simulink library "FVT_lib"  (R2021b)
settings: Solver=VariableStepAuto  StartTime=0.0  StopTime=10.0  RelTol=1e-3
undefined symbols (not defined in the file): C_TASK_5MS_S, CANFDArray, ENUM_FAULTSTATE_FAIL, ENUM_FAULTSTATE_INDETERMINATE, ENUM_FAULTSTATE_PASS, EPSILON, FALSE, KHAL_CounterMAX_enum, KHAL_CounterMAXE2E_enum, LINArray, ONE_INT, TRUE, UNKNOWN, XX2KXX, ZERO_FLOAT, ZERO_INT
libraries: hdlsllib x41, simulink x24, hcu_lib x7
(part 3 of 3)

== system FVT_lib/hal/DDM_ESC5_CS&RC_Comparison/CRC8_Compare/DetectChange2 ==
  cnt : Inport
  Constant : Constant  OutDataTypeStr=boolean
  Data Type Conversion3 : DataTypeConversion  OutDataTypeStr=uint8
  Delay : Delay  DelayLength=1  InitialCondition=0
  Delay1 : Delay  DelayLength=1  InitialCondition=0
  Logical Operator : Logic  AllPortsSameDT=off  OutDataTypeStr=boolean
  Relational Operator : RelationalOperator  Operator=~=  OutDataTypeStr=boolean  RndMeth=Simplest
  InValid : Outport
  wires:
  Logical Operator/1 -> InValid/1
  Relational Operator/1 -> Logical Operator/1
  Delay1/1 -> Logical Operator/2
  Constant/1 -> Delay1/1
  cnt/1 -> Delay/1, Relational Operator/1
  Delay/1 -> Data Type Conversion3/1
  Data Type Conversion3/1 -> Relational Operator/2

== system FVT_lib/hal/DDM_ESC5_CS&RC_Comparison/CRC8_Compare/Subsystem ==
  RC : Inport
  RC_delay : Inport  Port=2
  Enable : EnablePort
  Equal1 : RelationalOperator  Operator===  OutDataTypeStr=boolean  RndMeth=Simplest
  RCErr : Outport
  wires:
  RC_delay/1 -> Equal1/2
  Equal1/1 -> RCErr/1
  RC/1 -> Equal1/1

== system FVT_lib/hal/DDM_ESC5_CS&RC_Comparison/CRC8_Compare/Timer ==
  note: /* output signal type is single */
  trigger : Inport
  reset : Inport  Port=2
  Ts : Inport  Port=3
  max_time : Inport  Port=4
  Constant1 : Constant  Value=ZERO_FLOAT  OutDataTypeStr=single
  GreaterThan : RelationalOperator  Operator=<=  OutDataTypeStr=boolean  RndMeth=Simplest
  Subtract2 : Sum
  Switch : Switch  Criteria=u2 > Threshold
  Switch1 : Switch  Criteria=u2 ~= 0
      settings: AttributesFormatString=<%<Criteria>>
  Switch2 : Switch  Criteria=u2 ~= 0
      settings: AttributesFormatString=<%<Criteria>>
  Unit Delay1 : UnitDelay  SampleTime=-1  HasFrameUpgradeWarning=on
      settings: AttributesFormatString=<initial = %<X0>>
  time : Outport
  wires:
  GreaterThan/1 -> Switch/2
  Subtract2/1 -> Switch2/1
  trigger/1 -> Switch2/2
  reset/1 -> Switch1/2
  Constant1/1 -> Switch1/1
  Switch1/1 -> Switch2/3
  Ts/1 -> Subtract2/2
  Switch2/1 -> GreaterThan/2, Switch/3
  Switch/1 -> Unit Delay1/1, time/1
  Unit Delay1/1 -> Switch1/3, [last_time]
  max_time/1 -> GreaterThan/1, Switch/1
  [last_time] -> Subtract2/1

== system FVT_lib/hal/DDM_ESC5_CS&RC_Comparison/CRC8_IfAction_Rx/If Action Subsystem ==
  Raw : Inport
  Action Port : ActionPort
  CRC8_Caculation : Subsystem
      mask help: MeasumentTrigerEvent
      mask Display: fprintf('CRC8');
  CRC8_Result : Outport
  wires:
  CRC8_Caculation/1(CRCout) -> CRC8_Result/1
  Raw/1 -> CRC8_Caculation/1(MsgData)

== system FVT_lib/hal/DDM_ESC5_CS&RC_Comparison/CRC8_IfAction_Rx/If Action Subsystem1 ==
  CAN_E2E_ID1 : Inport
  CAN_E2E_ID2 : Inport  Port=2
  Raw : Inport  Port=3
  Action Port : ActionPort
  CRC8_E2EProfile1 : Subsystem
      mask help: MeasumentTrigerEvent
      mask Display: fprintf('CRC8_E2EProfile1');
  Mux2 : Mux  Inputs=3
  CRC8_E2EResult : Outport
  wires:
  Mux2/1 -> CRC8_E2EProfile1/1(MsgData)
  CAN_E2E_ID1/1 -> Mux2/1
  CAN_E2E_ID2/1 -> Mux2/2
  Raw/1 -> Mux2/3
  CRC8_E2EProfile1/1(CRCout) -> CRC8_E2EResult/1

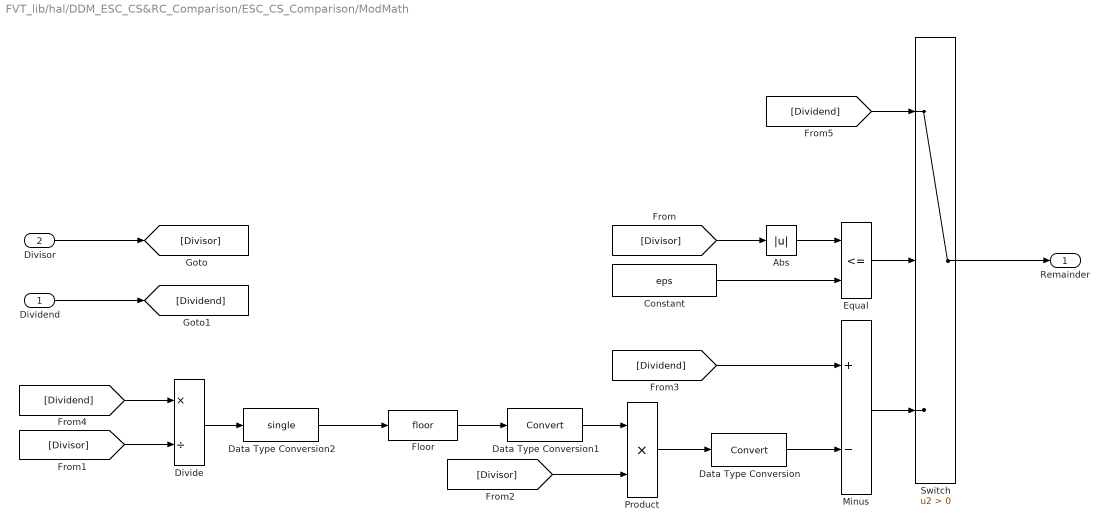
== system FVT_lib/hal/DDM_ESC_CS&RC_Comparison/ESC_CS_Comparison/ModMath ==
  Dividend : Inport
  Divisor : Inport  Port=2
  Abs : Abs
  Constant : Constant  Value=eps
  Data Type Conversion : DataTypeConversion
  Data Type Conversion1 : DataTypeConversion
  Data Type Conversion2 : DataTypeConversion  OutDataTypeStr=single
  Divide : Product  Inputs=*/
  Equal : RelationalOperator  Operator=<=  OutDataTypeStr=boolean  RndMeth=Simplest
  Floor : Rounding
  Minus : Sum  Inputs=+-
  Product : Product
  Switch : Switch  Criteria=u2 > Threshold
  Remainder : Outport
  wires:
  Divisor/1 -> [Divisor]
  Equal/1 -> Switch/2
  Constant/1 -> Equal/2
  [Dividend] -> Divide/1
  Switch/1 -> Remainder/1
  [Dividend] -> Switch/1
  Minus/1 -> Switch/3
  Data Type Conversion2/1 -> Floor/1
  Data Type Conversion/1 -> Minus/2
  [Dividend] -> Minus/1
  Dividend/1 -> [Dividend]
  Floor/1 -> Data Type Conversion1/1
  Data Type Conversion1/1 -> Product/1
  [Divisor] -> Divide/2
  Abs/1 -> Equal/1
  [Divisor] -> Product/2
  Divide/1 -> Data Type Conversion2/1
  Product/1 -> Data Type Conversion/1
  [Divisor] -> Abs/1

== system FVT_lib/hal/DDM_ESC_CS&RC_Comparison/RC_Compare/Counter ==
  note: /* Max Value of counter is 65535 */
  trigger : Inport
  reset : Inport  Port=2
  max_count : Inport  Port=3
  Constant1 : Constant  Value=ZERO_INT  OutDataTypeStr=uint16
  Constant2 : Constant  Value=uint16(1)  OutDataTypeStr=uint16
  Data Type Conversion : DataTypeConversion  OutDataTypeStr=uint16
  MinMax : MinMax  Inputs=2
  Saturation : Saturate  UpperLimit=65535  LowerLimit=0
      settings: AttributesFormatString=<upper = %<UpperLimit>>\n<lower = %<LowerLimit>>
  Subtract2 : Sum
  Switch1 : Switch  Criteria=u2 ~= 0
      settings: AttributesFormatString=<%<Criteria>>
  Switch2 : Switch  Criteria=u2 ~= 0
      settings: AttributesFormatString=<%<Criteria>>
  Unit Delay1 : UnitDelay  SampleTime=-1  HasFrameUpgradeWarning=on
      settings: AttributesFormatString=<initial = %<X0>>
  count : Outport
  wires:
  Data Type Conversion/1 -> Unit Delay1/1, count/1
  Subtract2/1 -> Switch2/1
  trigger/1 -> Switch2/2
  Switch2/1 -> Switch1/3
  Switch1/1 -> MinMax/2
  reset/1 -> Switch1/2
  Constant1/1 -> Switch1/1
  Constant2/1 -> Subtract2/2
  MinMax/1 -> Data Type Conversion/1
  Unit Delay1/1 -> [last_count], Switch2/3
  max_count/1 -> Saturation/1
  [last_count] -> Subtract2/1
  Saturation/1 -> MinMax/1

== system FVT_lib/hal/DDM_ESC_CS&RC_Comparison/RC_Compare/DetectChange2 ==
  cnt : Inport
  Constant : Constant  OutDataTypeStr=boolean
  Data Type Conversion3 : DataTypeConversion  OutDataTypeStr=uint8
  Delay : Delay  DelayLength=1  InitialCondition=0
  Delay1 : Delay  DelayLength=1  InitialCondition=0
  Logical Operator : Logic  AllPortsSameDT=off  OutDataTypeStr=boolean
  Relational Operator : RelationalOperator  Operator=~=  OutDataTypeStr=boolean  RndMeth=Simplest
  InValid : Outport
  wires:
  Logical Operator/1 -> InValid/1
  Relational Operator/1 -> Logical Operator/1
  Delay1/1 -> Logical Operator/2
  Constant/1 -> Delay1/1
  cnt/1 -> Delay/1, Relational Operator/1
  Delay/1 -> Data Type Conversion3/1
  Data Type Conversion3/1 -> Relational Operator/2

== system FVT_lib/hal/DDM_ESC_CS&RC_Comparison/RC_Compare/Subsystem ==
  RC : Inport
  RC_delay : Inport  Port=2
  Enable : EnablePort
  Equal1 : RelationalOperator  Operator===  OutDataTypeStr=boolean  RndMeth=Simplest
  RCErr : Outport
  wires:
  RC_delay/1 -> Equal1/2
  Equal1/1 -> RCErr/1
  RC/1 -> Equal1/1

== system FVT_lib/hal/DDM_ESC_CS&RC_Comparison/RC_Compare/Timer ==
  note: /* output signal type is single */
  trigger : Inport
  reset : Inport  Port=2
  Ts : Inport  Port=3
  max_time : Inport  Port=4
  Constant1 : Constant  Value=ZERO_FLOAT  OutDataTypeStr=single
  GreaterThan : RelationalOperator  Operator=<=  OutDataTypeStr=boolean  RndMeth=Simplest
  Subtract2 : Sum
  Switch : Switch  Criteria=u2 > Threshold
  Switch1 : Switch  Criteria=u2 ~= 0
      settings: AttributesFormatString=<%<Criteria>>
  Switch2 : Switch  Criteria=u2 ~= 0
      settings: AttributesFormatString=<%<Criteria>>
  Unit Delay1 : UnitDelay  SampleTime=-1  HasFrameUpgradeWarning=on
      settings: AttributesFormatString=<initial = %<X0>>
  time : Outport
  wires:
  GreaterThan/1 -> Switch/2
  Subtract2/1 -> Switch2/1
  trigger/1 -> Switch2/2
  reset/1 -> Switch1/2
  Constant1/1 -> Switch1/1
  Switch1/1 -> Switch2/3
  Ts/1 -> Subtract2/2
  Switch2/1 -> GreaterThan/2, Switch/3
  Switch/1 -> Unit Delay1/1, time/1
  Unit Delay1/1 -> Switch1/3, [last_time]
  max_time/1 -> GreaterThan/1, Switch/1
  [last_time] -> Subtract2/1

== system FVT_lib/inp/CAN_Msg_Validity_Process_template/CAN_Msg_Validity_Process/override_signal_m2  ==
  note: ONLY ONE ovrdflg (Service_ovrdflg and Cal_ovrdflg) can be valid
      | Set the priority of Service_ovrdflg higher than Cal_ovrdflg
      | In this way, the Cal_ovrd can be automatically disabled in production
  signal_raw : Inport
  cal_ovrdflg : Inport  Port=2
  cal_ovrdval : Inport  Port=3
  Switch1 : Switch  Criteria=u2 ~= 0  Threshold=0.5
  signal : Outport
  wires:
  cal_ovrdflg/1 -> Switch1/2  "cal_ovrdflg"
  cal_ovrdval/1 -> Switch1/1  "cal_ovrdval"
  signal_raw/1 -> Switch1/3  "signal_raw"
  Switch1/1 -> signal/1

== system FVT_lib/inp/ad_signal_template/ad_signal_process/override_signal_m2  ==
  note: ONLY ONE ovrdflg (Service_ovrdflg and Cal_ovrdflg) can be valid
      | Set the priority of Service_ovrdflg higher than Cal_ovrdflg
      | In this way, the Cal_ovrd can be automatically disabled in production
  note: When either service_ovrdflg or cal_ovrdflg is true, signal_valid_flg is set as TRUE
  signal_valid_flg_raw : Inport
  signal_raw : Inport  Port=2
  service_ovrdflg : Inport  Port=3
  service_ovrdval : Inport  Port=4
  cal_ovrdflg : Inport  Port=5
  cal_ovrdval : Inport  Port=6
  Data Type Duplicate : DataTypeDuplicate  NumInputPorts=5
  Logical Operator : Logic  Operator=OR  AllPortsSameDT=off  OutDataTypeStr=boolean
  Switch : Switch  Criteria=u2 ~= 0  Threshold=0.5
  Switch1 : Switch  Criteria=u2 ~= 0  Threshold=0.5
  Switch2 : Switch  Criteria=u2 ~= 0  Threshold=0.5
  True : Constant  Value=TRUE  OutDataTypeStr=boolean
  signal : Outport
  signal_valid_flg : Outport  Port=2
  wires:
  [cal_ovrdflg] -> Logical Operator/2
  [service_ovrdflg] -> Logical Operator/1
  Switch/1 -> Data Type Duplicate/5, signal/1  "signal"
  service_ovrdflg/1 -> [service_ovrdflg], Switch/2  "service_ovrdflg"
  cal_ovrdflg/1 -> [cal_ovrdflg], Switch1/2  "cal_ovrdflg"
  service_ovrdval/1 -> Data Type Duplicate/3, Switch/1  "service_ovrdval"
  cal_ovrdval/1 -> Data Type Duplicate/2, Switch1/1  "cal_ovrdval"
  signal_raw/1 -> Data Type Duplicate/1, Switch1/3  "signal_raw"
  Switch1/1 -> Data Type Duplicate/4, Switch/3
  Logical Operator/1 -> Switch2/2
  True/1 -> Switch2/1
  Switch2/1 -> signal_valid_flg/1  "signal_valid_flg"
  signal_valid_flg_raw/1 -> Switch2/3  "signal_valid_flg_raw"

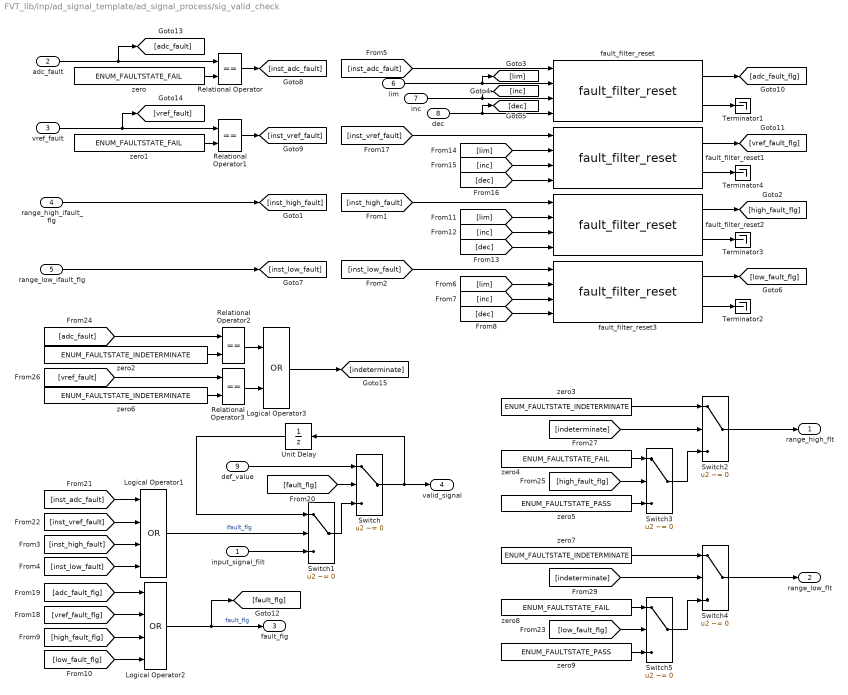
== system FVT_lib/inp/ad_signal_template/ad_signal_process/sig_valid_check ==
  input_signal_filt : Inport
  adc_fault : Inport  Port=2
  vref_fault : Inport  Port=3
  range_high_ifault_flg : Inport  Port=4
  range_low_ifault_flg : Inport  Port=5
  lim : Inport  Port=6
  inc : Inport  Port=7
  dec : Inport  Port=8
  def_value : Inport  Port=9
  Logical Operator1 : Logic  Operator=OR  Inputs=4  AllPortsSameDT=off  OutDataTypeStr=boolean
  Logical Operator2 : Logic  Operator=OR  Inputs=4  AllPortsSameDT=off  OutDataTypeStr=boolean
  Logical Operator3 : Logic  Operator=OR  AllPortsSameDT=off  OutDataTypeStr=boolean
  Relational Operator{,1..3} (4 alike) : RelationalOperator  Operator===  OutDataTypeStr=boolean  RndMeth=Nearest
  Switch{,1..5} (6 alike) : Switch  Criteria=u2 ~= 0
  Terminator{1..4} (4 alike) : Terminator
  Unit Delay : UnitDelay  SampleTime=-1
  fault_filter_reset{,1..3} (4 alike) : hcu_lib/Signal_Process_Blocks/fault_filter_reset
      settings: SourceProductName=HCU Relative Block Library
  zero{,1,4,8} (4 alike) : Constant  Tag=struct('comment',struct('text','','placement',1),'output',struct('width',1,'name','$S_$B','unit','','type','Int16','offset',0,'max',NaN,'min',NaN,'freeze',1,'lsb',1,'arb',0,'class','default','address','','description','','value','0','tolerance',1,'show',0),'date',731455.58675544)  Value=ENUM_FAULTSTATE_FAIL
  zero{2..3,6..7} (4 alike) : Constant  Tag=struct('comment',struct('text','','placement',1),'output',struct('width',1,'name','$S_$B','unit','','type','Int16','offset',0,'max',NaN,'min',NaN,'freeze',1,'lsb',1,'arb',0,'class','default','address','','description','','value','0','tolerance',1,'show',0),'date',731455.58675544)  Value=ENUM_FAULTSTATE_INDETERMINATE
  zero5 : Constant  Tag=struct('comment',struct('text','','placement',1),'output',struct('width',1,'name','$S_$B','unit','','type','Int16','offset',0,'max',NaN,'min',NaN,'freeze',1,'lsb',1,'arb',0,'class','default','address','','description','','value','0','tolerance',1,'show',0),'date',731455.58675544)  Value=ENUM_FAULTSTATE_PASS
  zero9 : Constant  Tag=struct('comment',struct('text','','placement',1),'output',struct('width',1,'name','$S_$B','unit','','type','Int16','offset',0,'max',NaN,'min',NaN,'freeze',1,'lsb',1,'arb',0,'class','default','address','','description','','value','0','tolerance',1,'show',0),'date',731455.58675544)  Value=ENUM_FAULTSTATE_PASS
  range_high_flt : Outport
  range_low_flt : Outport  Port=2
  fault_flg : Outport  Port=3
  valid_signal : Outport  Port=4
  wires:
  Switch4/1 -> range_low_flt/1
  [indeterminate] -> Switch4/2
  zero9/1 -> Switch5/3
  zero8/1 -> Switch5/1
  zero7/1 -> Switch4/1
  Switch5/1 -> Switch4/3
  [low_fault_flg] -> Switch5/2
  Logical Operator3/1 -> [indeterminate]
  [indeterminate] -> Switch2/2
  Relational Operator3/1 -> Logical Operator3/2
  Relational Operator2/1 -> Logical Operator3/1
  [vref_fault] -> Relational Operator3/1
  zero6/1 -> Relational Operator3/2
  Switch2/1 -> range_high_flt/1
  zero5/1 -> Switch3/3
  zero4/1 -> Switch3/1
  [adc_fault] -> Relational Operator2/1
  zero3/1 -> Switch2/1
  Switch3/1 -> Switch2/3
  [high_fault_flg] -> Switch3/2
  zero2/1 -> Relational Operator2/2
  [inst_low_fault] -> Logical Operator1/4
  [inst_high_fault] -> Logical Operator1/3
  [inst_vref_fault] -> Logical Operator1/2
  [inst_adc_fault] -> Logical Operator1/1
  Logical Operator2/1 -> [fault_flg], fault_flg/1  "fault_flg"
  [low_fault_flg] -> Logical Operator2/4
  [high_fault_flg] -> Logical Operator2/3
  [vref_fault_flg] -> Logical Operator2/2
  [adc_fault_flg] -> Logical Operator2/1
  fault_filter_reset2/1 -> [high_fault_flg]
  [inst_high_fault] -> fault_filter_reset2/1
  fault_filter_reset/1 -> [adc_fault_flg]
  [inst_adc_fault] -> fault_filter_reset/1
  fault_filter_reset1/1 -> [vref_fault_flg]
  fault_filter_reset1/2 -> Terminator4/1
  fault_filter_reset2/2 -> Terminator3/1
  [dec] -> fault_filter_reset1/4
  [inc] -> fault_filter_reset1/3
  [lim] -> fault_filter_reset1/2
  [inst_vref_fault] -> fault_filter_reset1/1
  [dec] -> fault_filter_reset2/4
  [inc] -> fault_filter_reset2/3
  [lim] -> fault_filter_reset2/2
  Relational Operator1/1 -> [inst_vref_fault]
  Relational Operator/1 -> [inst_adc_fault]
  vref_fault/1 -> [vref_fault], Relational Operator1/1
  zero1/1 -> Relational Operator1/2
  zero/1 -> Relational Operator/2
  adc_fault/1 -> [adc_fault], Relational Operator/1
  [dec] -> fault_filter_reset3/4
  [inc] -> fault_filter_reset3/3
  [lim] -> fault_filter_reset3/2
  fault_filter_reset3/2 -> Terminator2/1
  fault_filter_reset/2 -> Terminator1/1
  fault_filter_reset3/1 -> [low_fault_flg]
  range_low_ifault_flg/1 -> [inst_low_fault]
  Logical Operator1/1 -> Switch1/2  "ifault_flg"
  input_signal_filt/1 -> Switch1/3
  range_high_ifault_flg/1 -> [inst_high_fault]
  lim/1 -> fault_filter_reset/2, [lim]
  inc/1 -> fault_filter_reset/3, [inc]
  dec/1 -> fault_filter_reset/4, [dec]
  def_value/1 -> Switch/1
  Switch1/1 -> Switch/3
  Switch/1 -> valid_signal/1, Unit Delay/1
  [inst_low_fault] -> fault_filter_reset3/1
  [fault_flg] -> Switch/2
  Unit Delay/1 -> Switch1/1

== system FVT_lib/inp/ad_signal_template/ad_signal_process/signal_filter ==
  raw_input : Inport
  Tc : Inport  Port=2
  Ts : Inport  Port=3
  FirstOrderFilter1 : hcu_lib/Basic_Blocks/FirstOrderFilter
      settings: SourceProductName=HCU Relative Block Library
  IC : UnitDelay  Tag=struct('comment',struct('text','','placement',1),'logdata',struct('maxnumvals',inf,'plotchannels',[],'stepsize',0,'downsampling',1,'loggingmode',3,'channels',1),'output',struct('width',1,'name','$S_$B','unit','','type','Int16','offset',0,'max',NaN,'min',NaN,'freeze',1,'lsb',1,'arb',0,'class','default','address','','description','','autoscalingmode',1,'lowerheadroom',1,'upperheadroom',1,'headroomunit','bit','checkmin',0,'checkmax',0,'show',0,'initial','2'),'state',0,'dt','-1','date',731455.586925799)  SampleTime=-1
  Switch1 : Switch  Tag=struct('comment',struct('text','','placement',1),'logdata',struct('maxnumvals',inf,'plotchannels',[],'stepsize',0,'downsampling',1,'loggingmode',3,'channels',1),'output',struct('width',1,'name','$S_$B','unit','','type','Int32Bin15','offset',0,'max',65535,'min',-65536,'freeze',1,'lsb',2^-15,'arb',0,'class','default','address','','description','','autoscalingmode',1,'lowerheadroom',1,'upperheadroom',1,'headroomunit','bit','checkmin',0,'checkmax',0,'show',0),'threshold',struct('width',1,'name','$S_$B_threshold','unit','','type','Int16','offset',0,'max',NaN,'min',NaN,'freeze',1,'lsb',1,'arb',0,'class','default','address','','description','','value','1','scalar',0),'date',731455.58657044)  Threshold=0.5  InputSameDT=on
  zero : Constant  Tag=struct('comment',struct('text','','placement',1),'output',struct('width',1,'name','$S_$B','unit','','type','Int16','offset',0,'max',NaN,'min',NaN,'freeze',1,'lsb',1,'arb',0,'class','default','address','','description','','value','0','tolerance',1,'show',0),'date',731455.58675544)  Value=TRUE
  raw_input_filt : Outport
  wires:
  zero/1 -> IC/1
  raw_input/1 -> FirstOrderFilter1/1, Switch1/3
  Tc/1 -> FirstOrderFilter1/2
  Ts/1 -> FirstOrderFilter1/3
  IC/1 -> Switch1/2
  FirstOrderFilter1/1 -> Switch1/1
  Switch1/1 -> raw_input_filt/1

== system FVT_lib/inp/can_signal_template/can_signal_process/override_signal_m2  ==
  note: ONLY ONE ovrdflg (Service_ovrdflg and Cal_ovrdflg) can be valid
      | Set the priority of Service_ovrdflg higher than Cal_ovrdflg
      | In this way, the Cal_ovrd can be automatically disabled in production
  signal_raw : Inport
  cal_ovrdflg : Inport  Port=2
  cal_ovrdval : Inport  Port=3
  Switch1 : Switch  Criteria=u2 ~= 0  Threshold=0.5
  signal : Outport
  wires:
  Switch1/1 -> signal/1
  cal_ovrdflg/1 -> Switch1/2  "cal_ovrdflg"
  cal_ovrdval/1 -> Switch1/1  "cal_ovrdval"
  signal_raw/1 -> Switch1/3  "signal_raw"

== system FVT_lib/inp/can_signal_template/can_signal_process/signal validity checking ==
  new_signal : Inport
  new_signal_valid_flg : Inport  Port=2
  def_value : Inport  Port=3
  Logical Operator1 : Logic  Tag=struct('inputs','1','comment',struct('text','','placement',1),'logdata',struct('maxnumvals',inf,'plotchannels',[],'stepsize',0,'downsampling',1,'loggingmode',3,'channels',1),'operator','NOT','output',struct('class','default','type','Bool8','description','','address','','unit','','name','$S_$B'),'date',731430.46749816)  Operator=NOT  Inputs=1
  Switch : Switch  Criteria=u2 ~= 0
  Switch1 : Switch  Criteria=u2 ~= 0
  UnitDelay : UnitDelay  Tag=struct('comment',struct('text','','placement',1),'logdata',struct('maxnumvals',inf,'plotchannels',[],'stepsize',0,'downsampling',1,'loggingmode',3,'channels',1),'output',struct('width',1,'name','$S_$B','unit','','type','Int32Bin15','offset',0,'max',32767,'min',-32768,'freeze',1,'lsb',2^-16,'arb',0,'class','default','address','','description','','autoscalingmode',1,'lowerheadroom',1,'upperheadroom',1,'headroomunit','bit','checkmin',0,'checkmax',0,'show',0,'initial','0'),'state',0,'dt','-1','date',731401.644401968)  SampleTime=-1  HasFrameUpgradeWarning=on
  valid_signal : Outport
  wires:
  [ifault_flg] -> Switch/2  "ifault_flg"
  [ifault_flg] -> Switch1/2
  Logical Operator1/1 -> [ifault_flg]  "ifault_flg"
  new_signal/1 -> Switch1/3  "new_signal"
  Switch1/1 -> Switch/3
  UnitDelay/1 -> Switch1/1  "old_signal"
  new_signal_valid_flg/1 -> Logical Operator1/1  "new_signal_valid_flg"
  def_value/1 -> Switch/1  "def_value"
  Switch/1 -> UnitDelay/1, valid_signal/1  "valid_signal"

== system FVT_lib/inp/di_signal_template/digital_signal_process/AFL ==
  signal_in : Inport
  debounce_limit : Inport  Port=2
  debounce_inc : Inport  Port=3
  debounce_dec : Inport  Port=4
  Data Type Conversion : DataTypeConversion  OutDataTypeStr=uint8
  fault_acc : Stateflow chart  TreatAsAtomicUnit=on
  afl_fault : Outport
  wires:
  debounce_limit/1 -> fault_acc/2(max)
  signal_in/1 -> Data Type Conversion/1
  debounce_dec/1 -> fault_acc/4(dec)
  fault_acc/1(Signal_out) -> afl_fault/1  "fault_flg"
  debounce_inc/1 -> fault_acc/3(inc)
  Data Type Conversion/1 -> fault_acc/1(Signal_In)

== system FVT_lib/inp/di_signal_template/digital_signal_process/override_signal_m2  ==
  note: ONLY ONE ovrdflg (Service_ovrdflg and Cal_ovrdflg) can be valid
      | Set the priority of Service_ovrdflg higher than Cal_ovrdflg
      | In this way, the Cal_ovrd can be automatically disabled in production
  note: When either service_ovrdflg or cal_ovrdflg is true, signal_valid_flg is set as TRUE
  signal_valid_flg_raw : Inport
  signal_raw : Inport  Port=2
  service_ovrdflg : Inport  Port=3
  service_ovrdval : Inport  Port=4
  cal_ovrdflg : Inport  Port=5
  cal_ovrdval : Inport  Port=6
  Data Type Duplicate : DataTypeDuplicate  NumInputPorts=5
  Logical Operator : Logic  Operator=OR  AllPortsSameDT=off  OutDataTypeStr=boolean
  Switch : Switch  Criteria=u2 ~= 0  Threshold=0.5
  Switch1 : Switch  Criteria=u2 ~= 0  Threshold=0.5
  Switch2 : Switch  Criteria=u2 ~= 0  Threshold=0.5
  True : Constant  Value=TRUE  OutDataTypeStr=boolean
  signal : Outport
  signal_valid_flg : Outport  Port=2
  wires:
  [cal_ovrdflg] -> Logical Operator/2
  [service_ovrdflg] -> Logical Operator/1
  Switch/1 -> Data Type Duplicate/5, signal/1  "signal"
  service_ovrdflg/1 -> [service_ovrdflg], Switch/2  "service_ovrdflg"
  cal_ovrdflg/1 -> [cal_ovrdflg], Switch1/2  "cal_ovrdflg"
  service_ovrdval/1 -> Data Type Duplicate/3, Switch/1  "service_ovrdval"
  cal_ovrdval/1 -> Data Type Duplicate/2, Switch1/1  "cal_ovrdval"
  signal_raw/1 -> Data Type Duplicate/1, Switch1/3  "signal_raw"
  Switch1/1 -> Data Type Duplicate/4, Switch/3
  Logical Operator/1 -> Switch2/2
  True/1 -> Switch2/1
  Switch2/1 -> signal_valid_flg/1  "signal_valid_flg"
  signal_valid_flg_raw/1 -> Switch2/3  "signal_valid_flg_raw"

== system FVT_lib/outp/OverrideAndLimit/Signal_Limit/Limit ==
  input : Inport
  upper_limit : Inport  Port=2
  lower_limit : Inport  Port=3
  Saturation Dynamic : simulink/Discontinuities/Saturation Dynamic  OutMin=[]  OutMax=[]  OutDataTypeStr=Inherit: Same as second input  OutDataType=fixdt(1, 16)  OutScaling=2^-10  DoSatur=off
  out : Outport
  wires:
  input/1 -> Saturation Dynamic/2
  Saturation Dynamic/1 -> out/1
  upper_limit/1 -> Saturation Dynamic/1
  lower_limit/1 -> Saturation Dynamic/3

== system FVT_lib/outp/OverrideAndLimit/Signal_Override/override_signal_m2  ==
  signal_raw : Inport
  cal_ovrdflg : Inport  Port=2
  cal_ovrdval : Inport  Port=3
  Switch1 : Switch  Criteria=u2 ~= 0  Threshold=0.5
  signal : Outport
  wires:
  Switch1/1 -> signal/1  "signal"
  cal_ovrdflg/1 -> Switch1/2  "cal_ovrdflg"
  cal_ovrdval/1 -> Switch1/1  "cal_ovrdval"
  signal_raw/1 -> Switch1/3  "signal_raw"

== system FVT_lib/hal/DDM_CS&RC_Comparison/CRC8_IfAction_Rx/If Action Subsystem/CRC8_Caculation ==
  MsgData : Inport
  Data Type Conversion3 : DataTypeConversion  OutDataTypeStr=uint8
  Data Type Conversion4 : DataTypeConversion  OutDataTypeStr=uint8
  MATLAB Function : MATLAB Function  TreatAsAtomicUnit=on
  CRCout : Outport
  wires:
  MsgData/1 -> Data Type Conversion3/1
  Data Type Conversion3/1 -> MATLAB Function/1(msg_raw)
  MATLAB Function/1(CRC_Out) -> Data Type Conversion4/1
  Data Type Conversion4/1 -> CRCout/1

== system FVT_lib/hal/DDM_CS&RC_Comparison/CRC8_IfAction_Rx/If Action Subsystem1/CRC8_E2EProfile1 ==
  MsgData : Inport
  Data Type Conversion3 : DataTypeConversion  OutDataTypeStr=uint8
  Data Type Conversion4 : DataTypeConversion  OutDataTypeStr=uint8
  MATLAB Function : MATLAB Function  TreatAsAtomicUnit=on
  CRCout : Outport
  wires:
  Data Type Conversion4/1 -> CRCout/1
  MATLAB Function/1(CRC_Out) -> Data Type Conversion4/1
  Data Type Conversion3/1 -> MATLAB Function/1(msg_raw)
  MsgData/1 -> Data Type Conversion3/1

== system FVT_lib/hal/DDM_ESC5_CS&RC_Comparison/CRC8_IfAction_Rx/If Action Subsystem/CRC8_Caculation ==
  MsgData : Inport
  Data Type Conversion3 : DataTypeConversion  OutDataTypeStr=uint8
  Data Type Conversion4 : DataTypeConversion  OutDataTypeStr=uint8
  MATLAB Function : MATLAB Function  TreatAsAtomicUnit=on
  CRCout : Outport
  wires:
  Data Type Conversion4/1 -> CRCout/1
  MATLAB Function/1(CRC_Out) -> Data Type Conversion4/1
  Data Type Conversion3/1 -> MATLAB Function/1(msg_raw)
  MsgData/1 -> Data Type Conversion3/1

== system FVT_lib/hal/DDM_ESC5_CS&RC_Comparison/CRC8_IfAction_Rx/If Action Subsystem1/CRC8_E2EProfile1 ==
  MsgData : Inport
  Data Type Conversion3 : DataTypeConversion  OutDataTypeStr=uint8
  Data Type Conversion4 : DataTypeConversion  OutDataTypeStr=uint8
  MATLAB Function : MATLAB Function  TreatAsAtomicUnit=on
  CRCout : Outport
  wires:
  MsgData/1 -> Data Type Conversion3/1
  Data Type Conversion3/1 -> MATLAB Function/1(msg_raw)
  MATLAB Function/1(CRC_Out) -> Data Type Conversion4/1
  Data Type Conversion4/1 -> CRCout/1

== matlab function FVT_lib/hal/CRC8_IfAction_Tx/If Action Subsystem1/CRC8_E2EProfile1/MATLAB Function ==
  data: msg_raw input; CRC_Out output
function CRC_Out= fcn(msg_raw)

divisor = 0x1D;
messageLength = 8;
CRC_raw = uint8(0x00);

for i = 1:length(msg_raw(:,1))

    message = bitxor(CRC_raw,msg_raw(i));

    for k = 1:messageLength
        if bitget(message,8)
            message = bitshift(message,1);
            message = bitxor(message,divisor);
        else
            message = bitshift(message,1);
        end
    end
    CRC_raw = message;

end

CRC_Out = bitxor(CRC_raw,0x00);

== stateflow chart FVT_lib/hal/MsgTxController/Chart ==
  state TrigCounter
    en:
    counter = 0;
    counter++;
    (default) -> (junction 5)
    TrigCounter -> (junction 5) : {
        | counter++;
        | }
    (junction 5) -> (junction 6) [order 1] : [TxReq && (counter %% CycleCnt) == 0]
    (junction 5) -> (junction 7) [order 2]
    (junction 6) -> (junction 8) : {
        | TxTrigger;
        | counter = 0;
        | }
    (junction 8) -> (junction 7)
    (junction 7) -> (junction 34)
    (junction 34) -> (junction 33) [order 1] : [ !TxReq]
    (junction 34) -> (junction 35) [order 2]
    (junction 33) -> (junction 36) : {
        | counter = 0;
        | }
    (junction 36) -> (junction 35)
    (junction 35) -> (junction 44)
  data: TxReq input; CycleCnt input; counter local uint16
  events: TxTrigger output FUNCTION_CALL_EVENT

== stateflow chart FVT_lib/hal/LIN_Scheduler/Chart1 ==
  state Scheduler
    en:
    counter = 0;
    GoCyclic = FALSE;
    (default) -> (junction 36)
    Scheduler -> (junction 36) : {
        | counter++;
        | }
    (junction 36) -> (junction 37) [order 1] : [(counter == FirstDelayCounter) && !GoCyclic] /*first  delay */
    (junction 36) -> (junction 30) [order 2]
    (junction 37) -> (junction 32) : {
        | trig_LINReq;
        | GoCyclic = TRUE;
        | counter = 0;
        | }
    (junction 32) -> (junction 30)
    (junction 30) -> (junction 25)
    (junction 25) -> (junction 24) [order 1] : [(counter == CycleCounter) && GoCyclic]
    (junction 25) -> (junction 22) [order 2]
    (junction 24) -> (junction 26) : {
        | trig_LINReq;
        | counter = 0;
        | }
    (junction 26) -> (junction 22)
  (default) -> Scheduler
  data: GoCyclic local double; FALSE parameter; TRUE parameter; counter local double; CycleCounter input; FirstDelayCounter input
  events: trig_LINReq output FUNCTION_CALL_EVENT

== stateflow chart FVT_lib/inp/di_signal_template/digital_signal_process/AFL/fault_acc ==
  (default) -> (junction 25)
  (junction 25) -> (junction 20)
  (junction 20) -> (junction 29) [order 2] : [Signal_In==FALSE]
  (junction 20) -> (junction 27) [order 1] : [Signal_In==TRUE]
  (junction 29) -> (junction 30) : {count-=dec;}
  (junction 20) -> (junction 24) [order 3]
  (junction 27) -> (junction 28) : {count+=inc;}
  (junction 30) -> (junction 24)
  (junction 28) -> (junction 24)
  (junction 24) -> (junction 21)
  (junction 21) -> (junction 31) [order 2] : [count <= 0]
  (junction 21) -> (junction 33) [order 1] : [count >= max]
  (junction 31) -> (junction 32) : {count = 0;
      | Signal_out=FALSE;}
  (junction 21) -> (junction 22) [order 3]
  (junction 33) -> (junction 34) : {count = max;
      | Signal_out = TRUE;}
  (junction 32) -> (junction 22)
  (junction 34) -> (junction 22)
  (junction 22) -> (junction 26)
  (junction 26) -> (junction 23)
  data: Signal_In input; max input; inc input uint8; dec input uint8; Signal_out output boolean =0; count local int16 =0; TRUE parameter boolean; FALSE parameter boolean

== stateflow chart FVT_lib/hal/MsgTxController_Event/Chart ==
  state TrigCounter
    (default) -> (junction 5)
    TrigCounter -> (junction 5)
    (junction 5) -> (junction 6) [order 1] : [TxReq && EventReq]
    (junction 5) -> (junction 7) [order 2]
    (junction 6) -> (junction 8) : {
        | TxTrigger;
        | }
    (junction 8) -> (junction 7)
    (junction 7) -> (junction 21)
  data: TxReq input; EventReq input
  events: TxTrigger output FUNCTION_CALL_EVENT

== matlab function FVT_lib/hal/CRC8_E2EProfile1/MATLAB Function ==
  data: msg_raw input; CRC_Out output
function CRC_Out= fcn(msg_raw)

divisor = 0x1D;
messageLength = 8;
CRC_raw = uint8(0x00);

for i = 1:length(msg_raw(:,1))

    message = bitxor(CRC_raw,msg_raw(i));

    for k = 1:messageLength
        if bitget(message,8)
            message = bitshift(message,1);
            message = bitxor(message,divisor);
        else
            message = bitshift(message,1);
        end
    end
    CRC_raw = message;

end

CRC_Out = bitxor(CRC_raw,0x00);

== matlab function FVT_lib/hal/CRC8_Caculation/MATLAB Function ==
  data: msg_raw input; CRC_Out output
function CRC_Out= fcn(msg_raw)

divisor = 0x1D;
messageLength = 8;
CRC_raw = uint8(0xFF);

for i = 1:length(msg_raw(:,1))

    message = bitxor(CRC_raw,msg_raw(i));

    for k = 1:messageLength
        if bitget(message,8)
            message = bitshift(message,1);
            message = bitxor(message,divisor);
        else
            message = bitshift(message,1);
        end
    end
    CRC_raw = message;

end

CRC_Out = bitxor(CRC_raw,0xFF);

== stateflow chart FVT_lib/hal/MessageRollingCounter/Scheduler ==
  (default) -> (junction 1) [order 1] : {
      | counter = 0;
      | }
  (default) -> (junction 1) [order 2] : {
      | counter++;
      | }
  (junction 1) -> (junction 43) [order 1] : [(counter%%counter_max) == 0]
  (junction 1) -> (junction 5) [order 2]
  (junction 43) -> (junction 9) : {
      | trig_counter;
      | counter = 0;
      | }
  (junction 9) -> (junction 5)
  data: counter local uint16 size=1; counter_max input uint16
  events: trig_counter output FUNCTION_CALL_EVENT

== matlab function FVT_lib/hal/DDM_ESC5_CS&RC_Comparison/CRC8_IfAction_Rx/If Action Subsystem/CRC8_Caculation/MATLAB Function ==
  data: msg_raw input; CRC_Out output
function CRC_Out= fcn_DDM_ESC5_nonE2E_Comparison(msg_raw)

divisor = 0x2F;
messageLength = 8;
CRC_raw = uint8(0xFF);

for i = 1:length(msg_raw(:,1))

    message = bitxor(CRC_raw,msg_raw(i));

    for k = 1:messageLength
        if bitget(message,8)
            message = bitshift(message,1);
            message = bitxor(message,divisor);
        else
            message = bitshift(message,1);
        end
    end
    CRC_raw = message;

end

CRC_Out = bitxor(CRC_raw,0xFF);

== matlab function FVT_lib/hal/DDM_ESC5_CS&RC_Comparison/CRC8_IfAction_Rx/If Action Subsystem1/CRC8_E2EProfile1/MATLAB Function ==
  data: msg_raw input; CRC_Out output
function CRC_Out= fcn_DDM_ESC5_E2E_Comparison(msg_raw)

divisor = 0x2F;
messageLength = 8;
CRC_raw = uint8(0x00);

for i = 1:length(msg_raw(:,1))

    message = bitxor(CRC_raw,msg_raw(i));

    for k = 1:messageLength
        if bitget(message,8)
            message = bitshift(message,1);
            message = bitxor(message,divisor);
        else
            message = bitshift(message,1);
        end
    end
    CRC_raw = message;

end

CRC_Out = bitxor(CRC_raw,0x00);

== matlab function FVT_lib/hal/CRC8_IfAction_Tx/If Action Subsystem/CRC8_Caculation/MATLAB Function ==
  data: msg_raw input; CRC_Out output
function CRC_Out= fcn(msg_raw)

divisor = 0x1D;
messageLength = 8;
CRC_raw = uint8(0xFF);

for i = 1:length(msg_raw(:,1))

    message = bitxor(CRC_raw,msg_raw(i));

    for k = 1:messageLength
        if bitget(message,8)
            message = bitshift(message,1);
            message = bitxor(message,divisor);
        else
            message = bitshift(message,1);
        end
    end
    CRC_raw = message;

end

CRC_Out = bitxor(CRC_raw,0xFF);

== matlab function FVT_lib/hal/DDM_CS&RC_Comparison/CRC8_IfAction_Rx/If Action Subsystem/CRC8_Caculation/MATLAB Function ==
  data: msg_raw input; CRC_Out output
function CRC_Out= fcn_DDM_nonE2E_Comparison(msg_raw)

divisor = 0x1D;
messageLength = 8;
CRC_raw = uint8(0xFF);

for i = 1:length(msg_raw(:,1))

    message = bitxor(CRC_raw,msg_raw(i));

    for k = 1:messageLength
        if bitget(message,8)
            message = bitshift(message,1);
            message = bitxor(message,divisor);
        else
            message = bitshift(message,1);
        end
    end
    CRC_raw = message;

end

CRC_Out = bitxor(CRC_raw,0xFF);

== matlab function FVT_lib/hal/DDM_CS&RC_Comparison/CRC8_IfAction_Rx/If Action Subsystem1/CRC8_E2EProfile1/MATLAB Function ==
  data: msg_raw input; CRC_Out output
function CRC_Out= fcn_DDM_E2E_Comparison(msg_raw)

divisor = 0x1D;
messageLength = 8;
CRC_raw = uint8(0x00);

for i = 1:length(msg_raw(:,1))

    message = bitxor(CRC_raw,msg_raw(i));

    for k = 1:messageLength
        if bitget(message,8)
            message = bitshift(message,1);
            message = bitxor(message,divisor);
        else
            message = bitshift(message,1);
        end
    end
    CRC_raw = message;

end

CRC_Out = bitxor(CRC_raw,0x00);

== stateflow chart FVT_lib/hal/MsgTxController_CE/Chart ==
  state TrigCounter
    en:
    counter = 0;
    counter++;
    (default) -> (junction 5)
    TrigCounter -> (junction 5) : {
        | counter++;
        | CycleTriggerred = FALSE;
        | }
    (junction 5) -> (junction 6) [order 1] : [TxReq && (counter %% CycleCnt) == 0]
    (junction 5) -> (junction 7) [order 2]
    (junction 6) -> (junction 8) : {
        | TxTrigger;
        | counter = 0;
        | CycleTriggerred =TRUE;
        | }
    (junction 8) -> (junction 7)
    (junction 7) -> (junction 34)
    (junction 34) -> (junction 38) [order 1] : [TxReq && EventReq && !CycleTriggerred]
    (junction 34) -> (junction 36) [order 2]
    (junction 38) -> (junction 40) : {
        | TxTrigger;
        | }
    (junction 40) -> (junction 36)
    (junction 36) -> (junction 21)
    (junction 21) -> (junction 23) [order 1] : [ !TxReq]
    (junction 21) -> (junction 22) [order 2]
    (junction 23) -> (junction 20) : {
        | counter = 0;
        | }
    (junction 20) -> (junction 22)
    (junction 22) -> (junction 31)
  data: TxReq input; EventReq input; CycleCnt input; counter local uint16; CycleTriggerred local boolean; FALSE parameter; TRUE parameter
  events: TxTrigger output FUNCTION_CALL_EVENT
